simulink model "Modelo_NL_LTI"  (R2023b)
settings: Solver=VariableStepAuto  StartTime=0  StopTime=1  MaxStep=1e-4  RelTol=1e-3
values from neighbouring files (symbols this model uses):
  Ld = 6.6e-3    (= 0.0066)    [constantes.m]
  Lq = 5.8e-3    (= 0.0058)    [constantes.m]
  P_p = 3    [constantes.m]
settings Model: Creator=rodri  LastModifiedBy=nahue

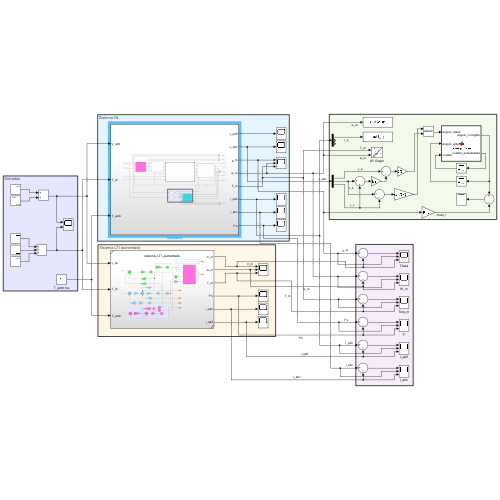
[thumbnail: Simulink's stored preview of the top-level diagram]
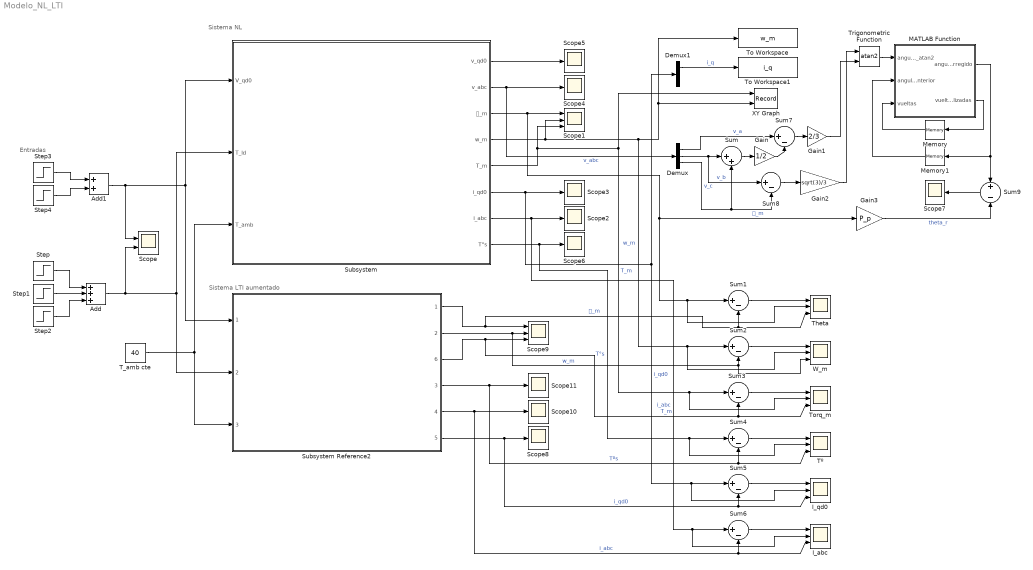
== system Modelo_NL_LTI ==
  note: Entradas
  note: Sistema LTI aumentado
  note: Sistema NL
  Add : Sum  Inputs=+++
  Add1 : Sum
  Demux : Demux  Outputs=3
  Demux1 : Demux  Outputs=3
  Gain : Gain  Gain=1/2
  Gain1 : Gain  Gain=2/3
  Gain2 : Gain  Gain=sqrt(3)/3
  Gain3 : Gain  Gain=P_p
  I_abc : Scope  NumInputPorts=3
  I_qd0 : Scope  NumInputPorts=3
  MATLAB Function : MATLAB Function  TreatAsAtomicUnit=on
  Memory : Memory
  Memory1 : Memory
  Scope : Scope  NumInputPorts=2
  Scope1 : Scope  NumInputPorts=3
  Scope{2..8,10..11} (9 alike) : Scope
  Scope9 : Scope  NumInputPorts=3
  Step : Step  Time=0.3  After=6.28  SampleTime=0.05
  Step1 : Step  Time=0.5  After=-6.28*2  SampleTime=0.05
  Step2 : Step  Time=0.9  After=6.28  SampleTime=0.05
  Step3 : Step  Time=0.1  After=19.596  SampleTime=0.05
  Step4 : Step  Time=0.7  After=-19.596  SampleTime=0.05
  Subsystem : Subsystem
  Subsystem Reference2 : Subsystem  ReferencedSubsystem=sistema_LTI_aumentado
      settings: PortSchema="{\"entries\":[{\"content\":{\"sides\":[{\"content\":{\"connectorIds\":[\"In1\",\"In2\",\"In3\"]},\"type\":\"ConnectorPlacement.EquallySpacedRectSide\",\"uuid\":\"a9fd203c-ee17-4a6f-9e49-b32a3c269841\"},{\"content\":{\"connectorIds\":[\"Out1\",\"Out2\",\"Out6\",\"Out3\",\"Out4\",\"Out5\"],\"side\":\"RIGHT\"},\"type\":\"ConnectorPlacement.EquallySpacedRectSide\",\"uuid\":\"bfddeaa7-7e9a-4fa0-b9ed-acae47f219cd\"},{\"content\":{\"side\":\"TOP\"},\"type\":\"ConnectorPlacement.EquallySpacedRectSide\",\"uuid\":\"01d68b23-e98f-4920-a18d-a9ccf9d9987a\"}]},\"type\":\"ConnectorPlacement.EquallySpacedConnector\",\"uuid\":\"92ceb62a-c405-4175-b2fa-7bbb7bcd3818\"}],\"packageUris\":[\"http://schema.mathworks.com/mf0/Connector/R2020b\"],\"version\":\"1.0\"}"
  Sum : Sum  Inputs=|++
  Sum{1..8} (8 alike) : Sum  Inputs=|+-
  Sum9 : Sum  Inputs=+-
  T_amb cte : Constant  Value=40
  Theta : Scope  NumInputPorts=3
  To Workspace : ToWorkspace  VariableName=w_m  SaveFormat=Timeseries  SampleTime=-1
  To Workspace1 : ToWorkspace  VariableName=i_q  SaveFormat=Timeseries  SampleTime=-1
  Torq_m : Scope  NumInputPorts=3
  Trigonometric Function : Trigonometry  Operator=atan2
  Tº : Scope  NumInputPorts=3
  W_m : Scope  NumInputPorts=3
  XY Graph : Record  FileSettingsInternal="{\"entries\":[{\"content\":{\"excelSettings\":{\"content\":{},\"type\":\"Streamout.ExcelSettings\"}},\"type\":\"Streamout.FileSettingStorage\",\"uuid\":\"\"}],\"packageUris\":[\"http:\\/\\/schema.mathworks.com\\/mf0\\/streamout_blocks\\/R2020a\"],\"version\":\"1.0\"}"  Layout=[1 1]  SignalsInternal="{\"entries\":[{\"content\":{\"signals\":[{\"content\":{\"blockPath\":[],\"dimensions\":[1],\"domain\":\"\",\"lineColor\":\"#a2142f\",\"plots\":[1],\"port\":1,\"signalID\":17,\"signalName\":\"T_m\"},\"type\":\"RecordBlkView.Signal\",\"uuid\":\"\"},{\"content\":{\"blockPath\":[],\"dimensions\":[1],\"domain\":\"\",\"lineColor\":\"#139fff\",\"plots\":[1],\"port\":2,\"signalID\":20,\"signalName\":\"w_m\"},\"type\":\"RecordBlkView.Signal\",\"uuid\":\"\"}]},\"type\":\"RecordBlkView.InputSignals\",\"uuid\":\"\"}],\"packageUris\":[\"http:\\/\\/schema.mathworks.com\\/mf0\\/streamout_blocks\\/R2020a\"],\"version\":\"1.0\"}"  VisualizationBindings="{\"xyplotplugin\":{\"info\":[{\"series\":[{\"bindingParametersList\":[{\"parameter\":\"X-Axis\",\"signalID\":17,\"signalName\":\"T_m\"},{\"parameter\":\"Y-Axis\",\"signalID\":20,\"signalName\":\"w_m\"}],\"seriesID\":11075}],\"subplotID\":1}]}}"  CompatibilityTag=XY
  wires:
  T_amb cte/1 -> Subsystem/3(T_amb), Subsystem Reference2/3
  Add1/1 -> Subsystem/1(V_qd0), Subsystem Reference2/1, Scope/1
  Step/1 -> Add/1
  Subsystem Reference2/1 -> Scope9/1, Sum1/2, Theta/3  "𝜃_m"
  Subsystem Reference2/2 -> W_m/3, Sum2/2, Scope9/2  "w_m"
  Subsystem Reference2/3 -> Scope11/1, Sum4/2, Tº/3  "Tºs"
  Subsystem Reference2/5 -> Sum5/2, I_qd0/3, Scope8/1  "i_qd0"
  Subsystem Reference2/6 -> Sum3/2, Torq_m/3, Scope9/3  "T_m"
  Subsystem Reference2/4 -> I_abc/3, Sum6/2, Scope10/1  "i_abc"
  Sum1/1 -> Theta/1
  Sum2/1 -> W_m/1
  Sum3/1 -> Torq_m/1
  Sum4/1 -> Tº/1
  Sum5/1 -> I_qd0/1
  Sum6/1 -> I_abc/1
  Add/1 -> Subsystem/2(T_ld), Subsystem Reference2/2, Scope/2
  Step4/1 -> Add1/2
  Step1/1 -> Add/2
  Step2/1 -> Add/3
  Step3/1 -> Add1/1
  Subsystem/6(i_qd0) -> Scope3/1, I_qd0/2, Sum5/1, Demux1/1  "i_qd0"
  Subsystem/7(i_abc) -> Scope2/1, I_abc/2, Sum6/1  "i_abc"
  Subsystem/1(v_qd0) -> Scope5/1
  Subsystem/2(v_abc) -> Demux/1, Scope4/1  "v_abc"
  Subsystem/3(𝜃_m) -> Scope1/1, Theta/2, Sum1/1, Gain3/1  "𝜃_m"
  Subsystem/4(w_m) -> Scope1/2, To Workspace/1, XY Graph/2, W_m/2, Sum2/1  "w_m"
  Subsystem/5(T_m) -> Scope1/3, XY Graph/1, Torq_m/2, Sum3/1  "T_m"
  Subsystem/8(T°s) -> Scope6/1, Tº/2, Sum4/1  "T°s"
  Demux1/1 -> To Workspace1/1  "i_q"
  Demux/1 -> Sum7/1  "v_a"
  Demux/2 -> Sum8/1, Sum/1  "v_b"
  Demux/3 -> Sum8/2, Sum/2  "v_c"
  Sum/1 -> Gain/1
  Gain/1 -> Sum7/2
  Sum7/1 -> Gain1/1
  Gain1/1 -> Trigonometric Function/2
  Sum8/1 -> Gain2/1
  Gain2/1 -> Trigonometric Function/1
  Gain3/1 -> Sum9/2  "theta_r"
  Sum9/1 -> Scope7/1
  MATLAB Function/2(vueltas_actualizadas) -> Memory/1
  Memory/1 -> MATLAB Function/3(vueltas)
  Memory1/1 -> MATLAB Function/2(angulo_anterior)
  MATLAB Function/1(angulo_corregido) -> Memory1/1, Sum9/1
  Trigonometric Function/1 -> MATLAB Function/1(angulo_atan2)

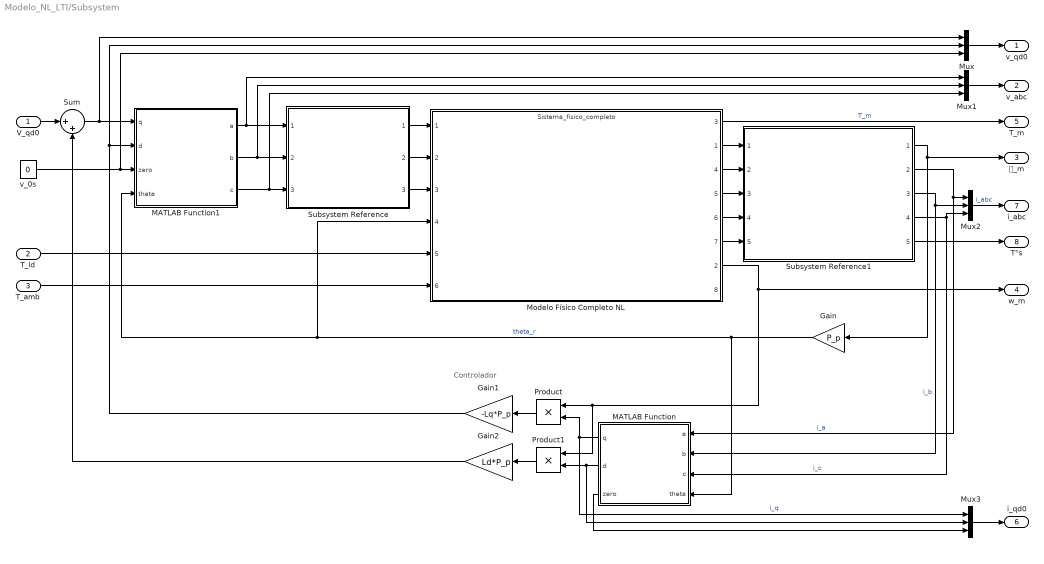
== system Modelo_NL_LTI/Subsystem ==
  note: Controlador
  V_qd0 : Inport
  T_ld : Inport  Port=2
  T_amb : Inport  Port=3
  Gain : Gain  Gain=P_p
  Gain1 : Gain  Gain=-Lq*P_p
  Gain2 : Gain  Gain=Ld*P_p
  MATLAB Function : MATLAB Function  TreatAsAtomicUnit=on
  MATLAB Function1 : MATLAB Function  TreatAsAtomicUnit=on
  Modelo Físico Completo NL : ModelReference  ModelNameDialog=Sistema_fisico_completo.slx  SimulationMode=Normal  ModelReferenceVersion=1.18
      settings: PortSchema="{\"entries\":[{\"content\":{\"sides\":[{\"content\":{\"connectorIds\":[\"In1\",\"In2\",\"In3\",\"In4\",\"In5\",\"In6\"]},\"type\":\"ConnectorPlacement.EquallySpacedRectSide\",\"uuid\":\"c38844a2-9b74-4da6-b9ce-d4868a84fb83\"},{\"content\":{\"connectorIds\":[\"Out3\",\"Out1\",\"Out4\",\"Out5\",\"Out6\",\"Out7\",\"Out2\",\"Out8\"],\"side\":\"RIGHT\"},\"type\":\"ConnectorPlacement.EquallySpacedRectSide\",\"uuid\":\"32cfc208-0644-4e1b-b9a9-83e6ff95cf9d\"},{\"content\":{\"side\":\"TOP\"},\"type\":\"ConnectorPlacement.EquallySpacedRectSide\",\"uuid\":\"4d8c9d59-309f-4ead-ae08-3f9c9c92e1b5\"}]},\"type\":\"ConnectorPlacement.EquallySpacedConnector\",\"uuid\":\"12663ecb-c0ca-4a2a-9423-b019766269d5\"}],\"packageUris\":[\"http://schema.mathworks.com/mf0/Connector/R2020b\"],\"version\":\"1.0\"}"
  Mux{,1..3} (4 alike) : Mux  Inputs=3
  Product : Product
  Product1 : Product
  Subsystem Reference : Subsystem  ReferencedSubsystem=modulador_tension
  Subsystem Reference1 : Subsystem  ReferencedSubsystem=sensores
  Sum : Sum  Inputs=|++
  v_0s : Constant  Value=0
  v_qd0 : Outport
  v_abc : Outport  Port=2
  𝜃_m : Outport  Port=3
  w_m : Outport  Port=4
  T_m : Outport  Port=5
  i_qd0 : Outport  Port=6
  i_abc : Outport  Port=7
  T°s : Outport  Port=8
  wires:
  T_ld/1 -> Modelo Físico Completo NL/5
  Subsystem Reference1/3 -> MATLAB Function/2(b), Mux2/2  "i_b"
  Modelo Físico Completo NL/6 -> Subsystem Reference1/4
  T_amb/1 -> Modelo Físico Completo NL/6
  MATLAB Function1/3(c) -> Subsystem Reference/3, Mux1/3
  Product/1 -> Gain1/1
  MATLAB Function1/1(a) -> Subsystem Reference/1, Mux1/1
  Modelo Físico Completo NL/1 -> Subsystem Reference1/1
  Modelo Físico Completo NL/7 -> Subsystem Reference1/5
  Subsystem Reference1/1 -> 𝜃_m/1, Gain/1
  Subsystem Reference/3 -> Modelo Físico Completo NL/3
  Subsystem Reference/1 -> Modelo Físico Completo NL/1
  Modelo Físico Completo NL/4 -> Subsystem Reference1/2
  MATLAB Function1/2(b) -> Subsystem Reference/2, Mux1/2
  Subsystem Reference1/5 -> T°s/1
  Gain1/1 -> MATLAB Function1/2(d), Mux/2
  Product1/1 -> Gain2/1
  v_0s/1 -> MATLAB Function1/3(zero), Mux/3
  V_qd0/1 -> Sum/1
  Sum/1 -> MATLAB Function1/1(q), Mux/1
  Subsystem Reference1/4 -> MATLAB Function/3(c), Mux2/3  "i_c"
  Subsystem Reference1/2 -> MATLAB Function/1(a), Mux2/1  "i_a"
  Mux1/1 -> v_abc/1
  Modelo Físico Completo NL/2 -> w_m/1, Product1/1, Product/1
  MATLAB Function/1(q) -> Product/2, Mux3/1  "i_q"
  Modelo Físico Completo NL/5 -> Subsystem Reference1/3
  Subsystem Reference/2 -> Modelo Físico Completo NL/2
  MATLAB Function/2(d) -> Mux3/2, Product1/2
  Gain/1 -> MATLAB Function/4(theta), Modelo Físico Completo NL/4, MATLAB Function1/4(theta)  "theta_r"
  MATLAB Function/3(zero) -> Mux3/3
  Mux/1 -> v_qd0/1
  Mux2/1 -> i_abc/1  "i_abc"
  Mux3/1 -> i_qd0/1
  Gain2/1 -> Sum/2
  Modelo Físico Completo NL/3 -> T_m/1  "T_m"

== matlab function Modelo_NL_LTI/Subsystem/MATLAB Function1 ==
  data: q input; a output; d input; zero input; theta input; b output; c output
function [a, b, c] = park_inversa(q, d, zero, theta)
    % Transformación de Park Inversa
    % Entradas:
    %   d, q, z: Coordenadas en el marco rotatorio
    %   theta: Ángulo en radianes
    % Salidas:
    %   a, b, c: Valores trifásicos reconstruidos
    
    % Constantes
    alpha = 2 * pi / 3; % Desplazamiento angular entre fases
    
    % Cálculo de valores trifásicos
    a = q * cos(theta) + d * sin(theta) + zero;
    b = q * cos(theta - alpha) + d * sin(theta - alpha) + zero;
    c = q * cos(theta + alpha) + d * sin(theta + alpha) + zero;
end

== matlab function Modelo_NL_LTI/Subsystem/MATLAB Function ==
  data: q output; a input; d output; b input; c input; theta input; zero output
function [q, d, zero] = park_directa(a, b, c, theta)
    % Transformación de Park Directa
    % Entradas:
    %   a, b, c: Valores trifásicos
    %   theta: Ángulo en radianes
    % Salidas:
    %   d, q, z: Coordenadas en el marco rotatorio
    
    % Constantes
    alpha = 2 * pi / 3; % Desplazamiento angular entre fases
    k = 2 / 3; % Escala para invarianza
    
    % Cálculo de coordenadas d, q, z
    q = k * (a * cos(theta) + b * cos(theta - alpha) + c * cos(theta + alpha));
    d = k * (a * sin(theta) + b * sin(theta - alpha) + c * sin(theta + alpha));
    zero = k * (a * 1/2 + b * 1/2 + c * 1/2);
end

== matlab function Modelo_NL_LTI/MATLAB Function ==
  data: angulo_atan2 input; angulo_corregido output; angulo_anterior input; vueltas input; vueltas_actualizadas output
function [angulo_corregido, vueltas_actualizadas] = corregir_fase(angulo_atan2, angulo_anterior, vueltas)
    delta = angulo_atan2 + vueltas * 2*pi - angulo_anterior;

    if delta < -pi
        vueltas = vueltas + 1;

    elseif delta > pi
        vueltas = vueltas - 1;
    end
    
    vueltas_actualizadas = vueltas;
    angulo_corregido = angulo_atan2 + vueltas_actualizadas * 2*pi;
end
